simulink model "Modelo_Sistema_Realimentado_Escalon"  (R2018b)
settings: Solver=FixedStepAuto  StartTime=0.0  StopTime=20.0  FixedStep=0.01  RelTol=0.001
settings Model: Creator=rafab  LastModifiedBy=rafab

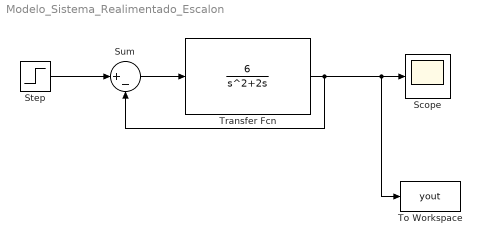
== system Modelo_Sistema_Realimentado_Escalon ==
  Scope : Scope
  Step : Step  SampleTime=0
  Sum : Sum  Inputs=|+-
  To Workspace : ToWorkspace  VariableName=yout  SampleTime=-1
      settings: Save2DSignal=2-D array (concatenate along first dimension)
  Transfer Fcn : TransferFcn  Numerator=[6]  Denominator=[1 2 0]
  wires:
  Transfer Fcn/1 -> To Workspace/1, Scope/1, Sum/2
  Sum/1 -> Transfer Fcn/1
  Step/1 -> Sum/1
